simulink model "TEP_Final_NoScript"  (R2024a)
settings: Solver=FixedStepAuto  StartTime=0.0  StopTime=10  FixedStep=1/3600  RelTol=1e-3
model workspace (MAT data in the model file):
  AD : Simulink.Parameter (value not decoded)
  AG : Simulink.Parameter (value not decoded)
  AH : Simulink.Parameter (value not decoded)
  AV : Simulink.Parameter (value not decoded)
  AVP : Simulink.Parameter (value not decoded)
  BCHL : Simulink.Parameter (value not decoded)
  BCHV : Simulink.Parameter (value not decoded)
  BD : Simulink.Parameter (value not decoded)
  BG : Simulink.Parameter (value not decoded)
  BH : Simulink.Parameter (value not decoded)
  BVP : Simulink.Parameter (value not decoded)
  CD : Simulink.Parameter (value not decoded)
  CG : Simulink.Parameter (value not decoded)
  CH : Simulink.Parameter (value not decoded)
  CVP : Simulink.Parameter (value not decoded)
  XMW : Simulink.Parameter (value not decoded)
  XNS : Simulink.Parameter (value not decoded)
  XNSE : Simulink.Parameter (value not decoded)
symbols that are objects in the model workspace (value not decoded): AD, AG, AH, AV, AVP, BD, BG, BH, BVP, CD, CG, CH, CVP, XMW, XNS, XNSE
undefined symbols (not defined in the file or in its folder): magnitude, msgbox, SETPT, XMEAS, XMV
libraries: mylib x360, dspindex x28
(part 3 of 14)

== system TEP_Final_NoScript/Separator/Stream 10 ==
  XST(I,10) : Inport
  TST(10) : Inport  Port=2  PortDimensions=1
  VPOS(6) : Inport  Port=3  PortDimensions=1
  Bus Creator : BusCreator  Inputs=6
  FCM(I,10) Component molar flow of Stream 10 lb-mol/h : Product
  FTM(10) : Product  Inputs=*/
  HST(10) Molar Enthalpy of Stream 10 MBtu/lb-mol : Subsystem
  ITY : Constant
  Subsystem : Subsystem
  XMWS(10) Molecular weight of Stream 10 lb/lb-mol : Subsystem
  Properties of Stream 10 : Outport  VectorParamsAs1DForOutWhenUnconnected=off
  wires:
  XMWS(10) Molecular weight of Stream 10 lb/lb-mol/1(XMWS(10)) -> FTM(10)/2
  FTM(10)/1 -> Bus Creator/4, FCM(I,10) Component molar flow of Stream 10 lb-mol/h/2  "FTM(10)"
  ITY/1 -> Bus Creator/6, HST(10) Molar Enthalpy of Stream 10 MBtu/lb-mol/1(ITY)  "Phase"
  XST(I,10)/1 -> Bus Creator/1, FCM(I,10) Component molar flow of Stream 10 lb-mol/h/1, HST(10) Molar Enthalpy of Stream 10 MBtu/lb-mol/3(XST(I,I)), XMWS(10) Molecular weight of Stream 10 lb/lb-mol/1(XST(I,10))  "XST(I;10)"
  HST(10) Molar Enthalpy of Stream 10 MBtu/lb-mol/1("H ") -> Bus Creator/3  "HST(10)"
  TST(10)/1 -> Bus Creator/2, HST(10) Molar Enthalpy of Stream 10 MBtu/lb-mol/2(T)  "TST(10)"
  FCM(I,10) Component molar flow of Stream 10 lb-mol/h/1 -> Bus Creator/5  "FCM(I;10)"
  Bus Creator/1 -> Properties of Stream 10/1
  VPOS(6)/1 -> Subsystem/1(VPOS(6))
  Subsystem/1(Out1) -> FTM(10)/1

== system TEP_Final_NoScript/Separator/Stream 11 ==
  XST(I,11) : Inport  PortDimensions=8
  TST(11) : Inport  Port=2  PortDimensions=1
  VPOS(7) : Inport  Port=3
  "   " : Constant  Value=100
  Bus Creator : BusCreator  Inputs=7
  FCM(I,11) Component molar flow of Stream 11 lb-mol/h : Product
  FTM(11) : Product  Inputs=**/
  HST(10) Molar Enthalpy of Stream 10 MBtu/lb-mol : Subsystem
  ITY : Constant  Value=0
  PTSL Pressure of Liquid From Separator mmHg : Subsystem
  VRNG(7) : Constant  Value=1500
  Properties of Stream 11 : Outport  VectorParamsAs1DForOutWhenUnconnected=off
  wires:
  FTM(11)/1 -> Bus Creator/4, FCM(I,11) Component molar flow of Stream 11 lb-mol/h/2  "FTM(11)"
  ITY/1 -> Bus Creator/6, HST(10) Molar Enthalpy of Stream 10 MBtu/lb-mol/1(ITY)  "Phase"
  XST(I,11)/1 -> PTSL Pressure of Liquid From Separator mmHg/1(XLS), FCM(I,11) Component molar flow of Stream 11 lb-mol/h/1, Bus Creator/1, HST(10) Molar Enthalpy of Stream 10 MBtu/lb-mol/3(XST(I,I))  "XST(I;11)"
  HST(10) Molar Enthalpy of Stream 10 MBtu/lb-mol/1("H ") -> Bus Creator/3  "HST(11)"
  TST(11)/1 -> PTSL Pressure of Liquid From Separator mmHg/2(TCS), Bus Creator/2, HST(10) Molar Enthalpy of Stream 10 MBtu/lb-mol/2(T)  "TST(11)"
  VPOS(7)/1 -> FTM(11)/1
  FCM(I,11) Component molar flow of Stream 11 lb-mol/h/1 -> Bus Creator/5  "FCM(I;11)"
  VRNG(7)/1 -> FTM(11)/2
  "   "/1 -> FTM(11)/3
  Bus Creator/1 -> Properties of Stream 11/1
  PTSL Pressure of Liquid From Separator mmHg/1(PTSL) -> Bus Creator/7  "PTSL"

== system TEP_Final_NoScript/Separator/Stream 9 ==
  TST(9) : Inport
  XTS(I,9) : Inport  Port=2
  VPOS(5) : Inport  Port=3
  "  " : Product  Inputs=*/
  Bus Creator : BusCreator  Inputs=7
  FCM(I,9) Component molar flow of Stream 9 lb-mol/h : Product
  FTM(9) : Product  Inputs=*/
  HST(9) Molar Enthalpy of Stream 9 MBtu/lb-mol : Subsystem
  "HST(9) " : Sum
  ITY : Constant
  Subsystem : Subsystem
  XMWS(9) Molecular weight of Stream 9 lb/lb-mol : Subsystem
  Properties of Stream 9 : Outport  VectorParamsAs1DForOutWhenUnconnected=off
  wires:
  XTS(I,9)/1 -> XMWS(9) Molecular weight of Stream 9 lb/lb-mol/1(XST(I,9)), FCM(I,9) Component molar flow of Stream 9 lb-mol/h/2, Bus Creator/1, HST(9) Molar Enthalpy of Stream 9 MBtu/lb-mol/3(XST(I,I))  "XST(I;9)"
  TST(9)/1 -> Bus Creator/2, HST(9) Molar Enthalpy of Stream 9 MBtu/lb-mol/2(T)  "TST(9)"
  XMWS(9) Molecular weight of Stream 9 lb/lb-mol/1(XMWS(9)) -> Bus Creator/6, FTM(9)/2  "XMWS(9)"
  FTM(9)/1 -> Bus Creator/4, "  "/2, FCM(I,9) Component molar flow of Stream 9 lb-mol/h/1  "FTM(9)"
  [CPDH] -> "  "/1
  HST(9) Molar Enthalpy of Stream 9 MBtu/lb-mol/1("H ") -> "HST(9) "/1
  "  "/1 -> "HST(9) "/2
  "HST(9) "/1 -> Bus Creator/3  "HST(9)"
  FCM(I,9) Component molar flow of Stream 9 lb-mol/h/1 -> Bus Creator/5  "FCM(I;9)"
  Bus Creator/1 -> Properties of Stream 9/1
  VPOS(5)/1 -> Subsystem/1(VPOS(5))
  Subsystem/1("FLMS ") -> FTM(9)/1
  ITY/1 -> Bus Creator/7, HST(9) Molar Enthalpy of Stream 9 MBtu/lb-mol/1(ITY)  "Phase"

== system TEP_Final_NoScript/Separator/TCS Initial Temperature in Separator °C  ==
  UTLS : Inport
  ETS : Inport  Port=2  PortDimensions=1
  XLS : Inport  Port=3  PortDimensions=8
  "AG(I) Coefficient A to determine Enthalpy MBtu/lb·°F " : Constant  Value=AG
  "AH(I) Coefficient A to determine Enthalpy MBtu/lb·°F " : Constant  Value=AH
  AV(I) Coefficient AV to determine Enthalpy MBtu/lb : Constant  Value=AV
  BG(I) Coefficient B to determine Enthalpy MBtu/lb·°F² : Constant  Value=BG
  BH(I) Coefficient B to determine Enthalpy MBtu/lb·°F² : Constant  Value=BH
  CG(I) Coefficient C to determine Enthalpy MBtu/lb·°F³ : Constant  Value=CG
  CH(I) Coefficient C to determine Enthalpy MBtu/lb·°F³ : Constant  Value=CH
  Delay : Delay  DelayLength=1  InitialCondition=0
  Display1 : Display
  ITY : Constant  Value=0
  MATLAB Function : MATLAB Function  TreatAsAtomicUnit=on
  "XMW(I) Molecular weight of components lb/lb-mol " : Constant  Value=XMW
  TCS : Outport  PortDimensions=1  VectorParamsAs1DForOutWhenUnconnected=off
  wires:
  MATLAB Function/1(TCS) -> Delay/1, TCS/1
  Delay/1 -> MATLAB Function/13("TCS ")
  "AG(I) Coefficient A to determine Enthalpy MBtu/lb·°F "/1 -> MATLAB Function/4(AG)
  AV(I) Coefficient AV to determine Enthalpy MBtu/lb/1 -> MATLAB Function/7(AV)
  MATLAB Function/2(J) -> Display1/1
  ETS/1 -> MATLAB Function/10(ETS)
  CH(I) Coefficient C to determine Enthalpy MBtu/lb·°F³/1 -> MATLAB Function/3(CH)
  UTLS/1 -> MATLAB Function/11(UTLS)
  ITY/1 -> MATLAB Function/12(ITY)
  "XMW(I) Molecular weight of components lb/lb-mol "/1 -> MATLAB Function/8(XMW)
  XLS/1 -> MATLAB Function/9(XLS)
  "AH(I) Coefficient A to determine Enthalpy MBtu/lb·°F "/1 -> MATLAB Function/1(AH)
  CG(I) Coefficient C to determine Enthalpy MBtu/lb·°F³/1 -> MATLAB Function/6(CG)
  BH(I) Coefficient B to determine Enthalpy MBtu/lb·°F²/1 -> MATLAB Function/2(BH)
  BG(I) Coefficient B to determine Enthalpy MBtu/lb·°F²/1 -> MATLAB Function/5(BG)

== system TEP_Final_NoScript/Separator/Total Vapour Component Holdup in Separator ==
  XVS : Inport
  VVS : Inport  Port=2
  Display9 : Display
  RG Universal Gas Constant ft³·mmHg/K·lb-mol : Constant  Value=998.9
  TKS Temperature in Separator K : Sum
  To Convert °C to K : Constant  Value=273.15
  "UCVS(I) Vapour Component Holdup in Separator lb-mol  " : Product  Inputs=**
  UTVS Total Vapour Component Holdup in Reactor lb-mol : Product  Inputs=**//
  wires:
  UTVS Total Vapour Component Holdup in Reactor lb-mol/1 -> "UCVS(I) Vapour Component Holdup in Separator lb-mol  "/1
  VVS/1 -> UTVS Total Vapour Component Holdup in Reactor lb-mol/2
  [PTS] -> UTVS Total Vapour Component Holdup in Reactor lb-mol/1
  XVS/1 -> "UCVS(I) Vapour Component Holdup in Separator lb-mol  "/2
  "UCVS(I) Vapour Component Holdup in Separator lb-mol  "/1 -> Display9/1
  RG Universal Gas Constant ft³·mmHg/K·lb-mol/1 -> UTVS Total Vapour Component Holdup in Reactor lb-mol/3
  TKS Temperature in Separator K/1 -> UTVS Total Vapour Component Holdup in Reactor lb-mol/4
  [TCS] -> TKS Temperature in Separator K/1
  To Convert °C to K/1 -> TKS Temperature in Separator K/2

== system TEP_Final_NoScript/Separator/Vapour Component Fraction in Separator ==
  PPS : Inport
  Bus Creator2 : BusCreator  Inputs=8
  Bus Selector1 : BusSelector  OutputSignals=PPS(1),PPS(2),PPS(3),PPS(4),PPS(5),PPS(6),PPS(7),PPS(8)
  XVS(1) : Product  Inputs=*/
  XVS(2) : Product  Inputs=*/
  XVS(3) : Product  Inputs=*/
  XVS(4) : Product  Inputs=*/
  XVS(5) : Product  Inputs=*/
  XVS(6) : Product  Inputs=*/
  XVS(7) : Product  Inputs=*/
  XVS(8) : Product  Inputs=*/
  XVS : Outport  PortDimensions=8  VectorParamsAs1DForOutWhenUnconnected=off
  wires:
  XVS(1)/1 -> Bus Creator2/1  "XVS(1)"
  Bus Selector1/5 -> XVS(5)/1  "<PPS(5)>"
  Bus Selector1/7 -> XVS(7)/1  "<PPS(7)>"
  Bus Selector1/6 -> XVS(6)/1  "<PPS(6)>"
  XVS(8)/1 -> Bus Creator2/8  "XVS(8)"
  Bus Selector1/8 -> XVS(8)/1  "<PPS(8)>"
  XVS(2)/1 -> Bus Creator2/2  "XVS(2)"
  [PTS] -> XVS(8)/2, XVS(7)/2, XVS(6)/2, XVS(5)/2, XVS(4)/2, XVS(3)/2, XVS(2)/2, XVS(1)/2
  Bus Selector1/2 -> XVS(2)/1  "<PPS(2)>"
  XVS(7)/1 -> Bus Creator2/7  "XVS(7)"
  Bus Selector1/4 -> XVS(4)/1  "<PPS(4)>"
  Bus Creator2/1 -> XVS/1
  XVS(4)/1 -> Bus Creator2/4  "XVS(4)"
  XVS(6)/1 -> Bus Creator2/6  "XVS(6)"
  Bus Selector1/3 -> XVS(3)/1  "<PPS(3)>"
  XVS(5)/1 -> Bus Creator2/5  "XVS(5)"
  PPS/1 -> Bus Selector1/1
  Bus Selector1/1 -> XVS(1)/1  "<PPS(1)>"
  XVS(3)/1 -> Bus Creator2/3  "XVS(3)"

== system TEP_Final_NoScript/Separator/Volume of Separator ==
  UTLS : Inport  PortDimensions=1
  XLS : Inport  Port=2  PortDimensions=8
  "DLS Molar Density of Liquids in Reactor lb-mol/ft³    " : Subsystem
  "VLS Liquid Volume in Separator ft³ " : Product  Inputs=*/
  VTS Total Volume of Separator ft³ : Constant  Value=3500
  VVS Vapour Volume in Separator ft³ : Sum  Inputs=+-
  VVS : Outport  VectorParamsAs1DForOutWhenUnconnected=off
  VLS : Outport  Port=2  VectorParamsAs1DForOutWhenUnconnected=off
  tag scope: DLS=global
  wires:
  "VLS Liquid Volume in Separator ft³ "/1 -> VLS/1, VVS Vapour Volume in Separator ft³/2
  VVS Vapour Volume in Separator ft³/1 -> VVS/1
  UTLS/1 -> "VLS Liquid Volume in Separator ft³ "/1
  VTS Total Volume of Separator ft³/1 -> VVS Vapour Volume in Separator ft³/1
  "DLS Molar Density of Liquids in Reactor lb-mol/ft³    "/1("DLS ") -> [DLS], "VLS Liquid Volume in Separator ft³ "/2
  XLS/1 -> "DLS Molar Density of Liquids in Reactor lb-mol/ft³    "/1(XLS)
  [TCS] -> "DLS Molar Density of Liquids in Reactor lb-mol/ft³    "/2(TCS)

== system TEP_Final_NoScript/Shut Down Procedure/Reactor Level to High ==
  VLR : Inport
  Assertion : Assertion  AssertionFailFcn=disp(sprintf('\nSimulation stoped.')), msgbox({'Plant Shutdown';'Reactor Level to High'}, 'Shutdown','error')  StopWhenAssertionFail=off
  Assertion block : mylib/Assertion block  SystemSampleTime=-1  VariantActivationTime=update diagram  AllowFlexibleInterface=on  Latency=0  AutoFrameSizeCalculation=off
      settings: SourceProductName=TEP Library
  Constant : Constant  Value=24
  Constant1 : Constant  Value=35.145
  Divide : Product  Inputs=*/
  Relational Operator : RelationalOperator  Operator=>  OutDataTypeStr=boolean  RndMeth=Simplest  InputSameDT=off
  ISD : Outport  VectorParamsAs1DForOutWhenUnconnected=off
  wires:
  Relational Operator/1 -> ISD/1, Assertion block/1
  Constant/1 -> Relational Operator/2
  Divide/1 -> Relational Operator/1
  VLR/1 -> Divide/1
  Constant1/1 -> Divide/2
  Assertion block/1 -> Assertion/1

== system TEP_Final_NoScript/Shut Down Procedure/Reactor Level to Low ==
  VLR : Inport
  Assertion : Assertion  AssertionFailFcn=disp(sprintf('\nSimulation stoped.')), msgbox({'Plant Shutdown';'Reactor Level to Low'}, 'Shutdown','error')  StopWhenAssertionFail=off
  Assertion block : mylib/Assertion block  SystemSampleTime=-1  VariantActivationTime=update diagram  AllowFlexibleInterface=on  Latency=0  AutoFrameSizeCalculation=off
      settings: SourceProductName=TEP Library
  Constant : Constant  Value=2
  Constant1 : Constant  Value=35.145
  Divide : Product  Inputs=*/
  Relational Operator : RelationalOperator  Operator=<  OutDataTypeStr=boolean  RndMeth=Simplest  InputSameDT=off
  ISD : Outport  VectorParamsAs1DForOutWhenUnconnected=off
  wires:
  Relational Operator/1 -> ISD/1, Assertion block/1
  Constant/1 -> Relational Operator/2
  Divide/1 -> Relational Operator/1
  VLR/1 -> Divide/1
  Constant1/1 -> Divide/2
  Assertion block/1 -> Assertion/1

== system TEP_Final_NoScript/Shut Down Procedure/Reactor Presssure to High ==
  " " : Sum  Inputs=+-
  "    " : Constant  Value=760
  "       " : Constant  Value=101.325
  Assertion : Assertion  AssertionFailFcn=disp(sprintf('\nSimulation stoped.')), msgbox({'Plant Shutdown';'Reactor Pressure to High'}, 'Shutdown','error')  StopWhenAssertionFail=off
  Assertion block : mylib/Assertion block  SystemSampleTime=-1  VariantActivationTime=update diagram  AllowFlexibleInterface=on  Latency=0  AutoFrameSizeCalculation=off
      settings: SourceProductName=TEP Library
  Constant : Constant  Value=3000
  Relational Operator : RelationalOperator  Operator=>  RndMeth=Simplest  InputSameDT=off
  XMEAS(7) : Product  Inputs=*/*
  ISD : Outport  VectorParamsAs1DForOutWhenUnconnected=off
  wires:
  XMEAS(7)/1 -> Relational Operator/1
  Relational Operator/1 -> ISD/1, Assertion block/1
  Constant/1 -> Relational Operator/2
  "       "/1 -> XMEAS(7)/3
  " "/1 -> XMEAS(7)/1
  [PTR] -> " "/1
  "    "/1 -> XMEAS(7)/2, " "/2
  Assertion block/1 -> Assertion/1

== system TEP_Final_NoScript/Shut Down Procedure/Reactor Temperature to High ==
  Assertion : Assertion  AssertionFailFcn=disp(sprintf('\nSimulation stoped.')), msgbox({'Plant Shutdown';'Reactor Temperature to High'}, 'Shutdown','error')  StopWhenAssertionFail=off
  Assertion block : mylib/Assertion block  SystemSampleTime=-1  VariantActivationTime=update diagram  AllowFlexibleInterface=on  Latency=0  AutoFrameSizeCalculation=off
      settings: SourceProductName=TEP Library
  Constant : Constant  Value=175
  Relational Operator : RelationalOperator  Operator=>  OutDataTypeStr=boolean  RndMeth=Simplest  InputSameDT=off
  ISD : Outport  VectorParamsAs1DForOutWhenUnconnected=off
  wires:
  [TCR] -> Relational Operator/1
  Relational Operator/1 -> ISD/1, Assertion block/1
  Constant/1 -> Relational Operator/2
  Assertion block/1 -> Assertion/1

== system TEP_Final_NoScript/Shut Down Procedure/Separator Level to High ==
  VLS : Inport
  Assertion : Assertion  AssertionFailFcn=disp(sprintf('\nSimulation stoped.')), msgbox({'Plant Shutdown';'Separator Level to High'}, 'Shutdown','error')  StopWhenAssertionFail=off
  Assertion block : mylib/Assertion block  SystemSampleTime=-1  VariantActivationTime=update diagram  AllowFlexibleInterface=on  Latency=0  AutoFrameSizeCalculation=off
      settings: SourceProductName=TEP Library
  Constant : Constant  Value=12
  Constant1 : Constant  Value=35.145
  Divide : Product  Inputs=*/
  Relational Operator : RelationalOperator  Operator=>  OutDataTypeStr=boolean  RndMeth=Simplest  InputSameDT=off
  ISD : Outport  VectorParamsAs1DForOutWhenUnconnected=off
  wires:
  Relational Operator/1 -> ISD/1, Assertion block/1
  Constant/1 -> Relational Operator/2
  Divide/1 -> Relational Operator/1
  VLS/1 -> Divide/1
  Constant1/1 -> Divide/2
  Assertion block/1 -> Assertion/1

== system TEP_Final_NoScript/Shut Down Procedure/Separator Level to Low ==
  VLS : Inport
  Assertion : Assertion  AssertionFailFcn=disp(sprintf('\nSimulation stoped.')), msgbox({'Plant Shutdown';'Separator Level to Low'}, 'Shutdown','error')  StopWhenAssertionFail=off
  Assertion block : mylib/Assertion block  SystemSampleTime=-1  VariantActivationTime=update diagram  AllowFlexibleInterface=on  Latency=0  AutoFrameSizeCalculation=off
      settings: SourceProductName=TEP Library
  Constant : Constant
  Constant1 : Constant  Value=35.145
  Divide : Product  Inputs=*/
  Relational Operator : RelationalOperator  Operator=<  OutDataTypeStr=boolean  RndMeth=Simplest  InputSameDT=off
  ISD : Outport  VectorParamsAs1DForOutWhenUnconnected=off
  wires:
  Relational Operator/1 -> ISD/1, Assertion block/1
  Constant/1 -> Relational Operator/2
  Divide/1 -> Relational Operator/1
  VLS/1 -> Divide/1
  Constant1/1 -> Divide/2
  Assertion block/1 -> Assertion/1

== system TEP_Final_NoScript/Shut Down Procedure/Stripper Level to High ==
  VLC : Inport
  Assertion : Assertion  AssertionFailFcn=disp(sprintf('\nSimulation stoped.')), msgbox({'Plant Shutdown';'Stripper Level to High'}, 'Shutdown','error')  StopWhenAssertionFail=off
  Assertion block : mylib/Assertion block  SystemSampleTime=-1  VariantActivationTime=update diagram  AllowFlexibleInterface=on  Latency=0  AutoFrameSizeCalculation=off
      settings: SourceProductName=TEP Library
  Constant : Constant  Value=8
  Constant1 : Constant  Value=35.145
  Divide : Product  Inputs=*/
  Relational Operator : RelationalOperator  Operator=>  OutDataTypeStr=boolean  RndMeth=Simplest  InputSameDT=off
  ISD : Outport  VectorParamsAs1DForOutWhenUnconnected=off
  wires:
  Relational Operator/1 -> ISD/1, Assertion block/1
  Constant/1 -> Relational Operator/2
  VLC/1 -> Divide/1
  Constant1/1 -> Divide/2
  Divide/1 -> Relational Operator/1
  Assertion block/1 -> Assertion/1

== system TEP_Final_NoScript/Shut Down Procedure/Stripper Level to Low ==
  VLC : Inport
  Assertion : Assertion  AssertionFailFcn=disp(sprintf('\nSimulation stoped.')), msgbox({'Plant Shutdown';'Stripper Level to Low'}, 'Shutdown','error')  StopWhenAssertionFail=off
  Assertion block : mylib/Assertion block  SystemSampleTime=-1  VariantActivationTime=update diagram  AllowFlexibleInterface=on  Latency=0  AutoFrameSizeCalculation=off
      settings: SourceProductName=TEP Library
  Constant : Constant
  Constant1 : Constant  Value=35.145
  Divide : Product  Inputs=*/
  Relational Operator : RelationalOperator  Operator=<  OutDataTypeStr=boolean  RndMeth=Simplest  InputSameDT=off
  ISD : Outport  VectorParamsAs1DForOutWhenUnconnected=off
  wires:
  Relational Operator/1 -> ISD/1, Assertion block/1
  Constant/1 -> Relational Operator/2
  Divide/1 -> Relational Operator/1
  VLC/1 -> Divide/1
  Constant1/1 -> Divide/2
  Assertion block/1 -> Assertion/1

== system TEP_Final_NoScript/Stripper/Heat transfer of stripper ==
  VPOS(9) : Inport
  "  " : Constant  Value=0
  Add : Sum
  Bus Selector : BusSelector  OutputSignals=signal1.TESUB8(9)
  Constant : Constant
  Constant2 : Constant  Value=100
  If : If  IfExpression=u1 < 100
  If Action Subsystem : Subsystem  TreatAsAtomicUnit=on
  If Action Subsystem1 : Subsystem  TreatAsAtomicUnit=on
  Merge : Merge
  Product : Product
  Subtract : Sum  Inputs=+-
  UAC : Product  Inputs=***/
  VRNG(9) : Constant  Value=0.03
  tag scope: QUC=global
  wires:
  Constant/1 -> Add/1
  Bus Selector/1 -> Add/2  "<TESUB8(9)>"
  VPOS(9)/1 -> UAC/1
  VRNG(9)/1 -> UAC/2
  Add/1 -> UAC/3
  Constant2/1 -> Subtract/1, UAC/4
  If/1 -> If Action Subsystem/Action
  Product/1 -> If Action Subsystem/1(In1)
  [TCC] -> Subtract/2, If/1
  If/2 -> If Action Subsystem1/Action
  "  "/1 -> If Action Subsystem1/1(In1)
  Subtract/1 -> Product/2
  UAC/1 -> Product/1
  If Action Subsystem/1(Out1) -> Merge/1
  If Action Subsystem1/1(Out1) -> Merge/2
  Merge/1 -> [QUC]
  [TESUB8] -> Bus Selector/1

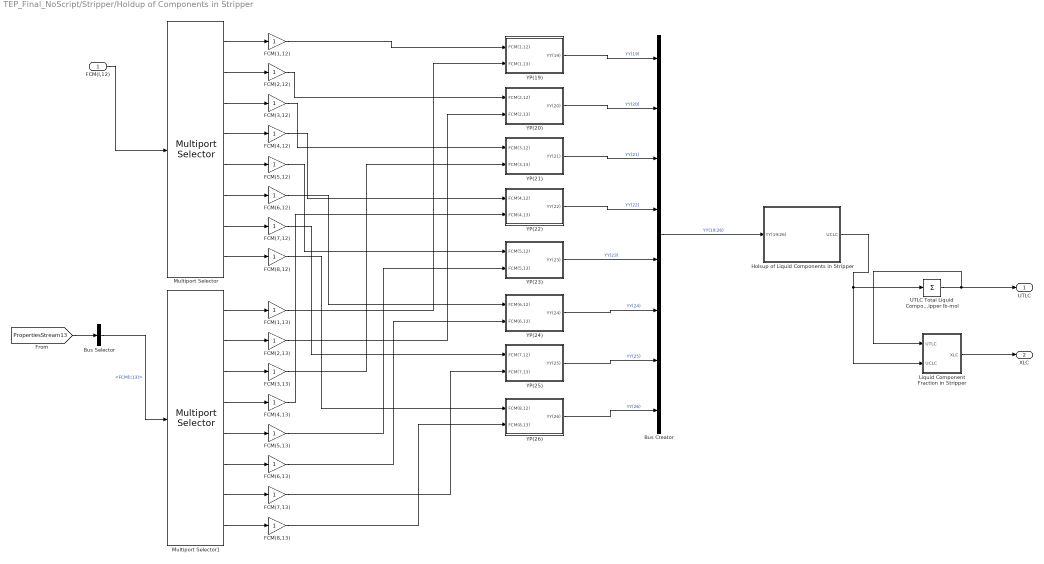
== system TEP_Final_NoScript/Stripper/Holdup of Components in Stripper ==
  "FCM(I,12) " : Inport
  Bus Creator : BusCreator  Inputs=8
  Bus Selector : BusSelector  OutputSignals=FCM(I;13)
  FCM(1,12) : Gain
  FCM(1,13) : Gain
  FCM(2,12) : Gain
  FCM(2,13) : Gain
  FCM(3,12) : Gain
  FCM(3,13) : Gain
  FCM(4,12) : Gain
  FCM(4,13) : Gain
  FCM(5,12) : Gain
  FCM(5,13) : Gain
  FCM(6,12) : Gain
  FCM(6,13) : Gain
  FCM(7,12) : Gain
  FCM(7,13) : Gain
  FCM(8,12) : Gain
  FCM(8,13) : Gain
  Holsup of Liquid Components in Stripper : Subsystem
  Liquid Component Fraction in Stripper : Subsystem
  Multiport Selector : dspindex/Multiport Selector  rowsOrCols=Rows  idxCellArray={ 1,2,3,4,5,6,7,8}  idxErrMode=Clip Index
  Multiport Selector1 : dspindex/Multiport Selector  rowsOrCols=Rows  idxCellArray={ 1,2,3,4,5,6,7,8}  idxErrMode=Clip Index
  UTLC Total Liquid Component holdup in Stripper lb-mol : Sum  Inputs=+
  YP(19) : Subsystem
  YP(20) : Subsystem
  YP(21) : Subsystem
  YP(22) : Subsystem
  YP(23) : Subsystem
  YP(24) : Subsystem
  YP(25) : Subsystem
  YP(26) : Subsystem
  UTLC : Outport  VectorParamsAs1DForOutWhenUnconnected=off
  XLC : Outport  Port=2  VectorParamsAs1DForOutWhenUnconnected=off
  wires:
  "FCM(I,12) "/1 -> Multiport Selector/1
  Multiport Selector/1 -> FCM(1,12)/1
  Multiport Selector/2 -> FCM(2,12)/1
  Multiport Selector/3 -> FCM(3,12)/1
  Multiport Selector/4 -> FCM(4,12)/1
  Multiport Selector/5 -> FCM(5,12)/1
  Multiport Selector/6 -> FCM(6,12)/1
  Multiport Selector/7 -> FCM(7,12)/1
  Multiport Selector/8 -> FCM(8,12)/1
  Multiport Selector1/1 -> FCM(1,13)/1
  Multiport Selector1/7 -> FCM(7,13)/1
  Multiport Selector1/2 -> FCM(2,13)/1
  Multiport Selector1/3 -> FCM(3,13)/1
  Multiport Selector1/5 -> FCM(5,13)/1
  Multiport Selector1/4 -> FCM(4,13)/1
  Multiport Selector1/8 -> FCM(8,13)/1
  Multiport Selector1/6 -> FCM(6,13)/1
  FCM(1,12)/1 -> YP(19)/1(FCM(1,12))
  YP(19)/1(YY(19)) -> Bus Creator/1  "YY(19)"
  YP(20)/1(YY(20)) -> Bus Creator/2  "YY(20)"
  YP(22)/1("YY(22)  ") -> Bus Creator/4  "YY(22)"
  YP(23)/1("YY(23)  ") -> Bus Creator/5  "YY(23)"
  YP(24)/1("YY(24)  ") -> Bus Creator/6  "YY(24)"
  YP(25)/1("YY(25)  ") -> Bus Creator/7  "YY(25)"
  YP(26)/1("YY(26)   ") -> Bus Creator/8  "YY(26)"
  FCM(1,13)/1 -> YP(19)/2(FCM(1,13))
  FCM(2,12)/1 -> YP(20)/1(FCM(2,12))
  FCM(3,12)/1 -> YP(21)/1(FCM(3,12))
  FCM(4,12)/1 -> YP(22)/1(FCM(4,12))
  FCM(5,12)/1 -> YP(23)/1(FCM(5,12))
  FCM(2,13)/1 -> YP(20)/2(FCM(2,13))
  FCM(3,13)/1 -> YP(21)/2(FCM(3,13))
  FCM(6,12)/1 -> YP(24)/1(FCM(6,12))
  FCM(7,12)/1 -> YP(25)/1(FCM(7,12))
  FCM(8,12)/1 -> YP(26)/1(FCM(8,12))
  FCM(4,13)/1 -> YP(22)/2(FCM(4,13))
  FCM(5,13)/1 -> YP(23)/2(FCM(5,13))
  FCM(6,13)/1 -> YP(24)/2(FCM(6,13))
  FCM(7,13)/1 -> YP(25)/2(FCM(7,13))
  FCM(8,13)/1 -> YP(26)/2(FCM(8,13))
  Bus Creator/1 -> Holsup of Liquid Components in Stripper/1(YY(19:26))  "YY(19:26)"
  Holsup of Liquid Components in Stripper/1(UCLC) -> Liquid Component Fraction in Stripper/2(UCLC), UTLC Total Liquid Component holdup in Stripper lb-mol/1
  YP(21)/1(YY(21)) -> Bus Creator/3  "YY(21)"
  UTLC Total Liquid Component holdup in Stripper lb-mol/1 -> Liquid Component Fraction in Stripper/1(UTLC), UTLC/1
  Liquid Component Fraction in Stripper/1(XLC) -> XLC/1
  [PropertiesStream13] -> Bus Selector/1
  Bus Selector/1 -> Multiport Selector1/1  "<FCM(I;13)>"

== system TEP_Final_NoScript/Stripper/Internal energy of stripper ==
  Properties of Stream 4 : Inport
  Properties of Stream 11 : Inport  Port=2
  Properties of Stream 5 : Inport  Port=3
  Add : Sum  Inputs=++--+
  Bus Selector : BusSelector  OutputSignals=HST(4),FTM(4)
  Bus Selector1 : BusSelector  OutputSignals=HST(11),FTM(11)
  Bus Selector2 : BusSelector  OutputSignals=HST(5),FTM(5)
  Bus Selector3 : BusSelector  OutputSignals=HST(13),FTM(13)
  Integration : mylib/Integration  SystemSampleTime=-1  VariantActivationTime=update diagram  AllowFlexibleInterface=on  Latency=0  AutoFrameSizeCalculation=off
      settings: SourceProductName=TEP Library
  Product{,1..3} (4 alike) : Product
  YY(27) : Constant  Value=0.3755297257
  "YY(27) " : Outport  VectorParamsAs1DForOutWhenUnconnected=off
  wires:
  Bus Selector/1 -> Product/1  "<HST(4)>"
  Bus Selector/2 -> Product/2  "<FTM(4)>"
  Bus Selector1/2 -> Product1/2  "<FTM(11)>"
  Bus Selector1/1 -> Product1/1  "<HST(11)>"
  Product/1 -> Add/1
  Product1/1 -> Add/2
  Integration/1 -> "YY(27) "/1
  YY(27)/1 -> Integration/2
  Add/1 -> Integration/1
  Bus Selector3/1 -> Product3/1  "<HST(13)>"
  Bus Selector2/2 -> Product2/2  "<FTM(5)>"
  Product2/1 -> Add/3
  Bus Selector3/2 -> Product3/2  "<FTM(13)>"
  Product3/1 -> Add/4
  Bus Selector2/1 -> Product2/1  "<HST(5)>"
  [QUC] -> Add/5
  Properties of Stream 4/1 -> Bus Selector/1
  Properties of Stream 11/1 -> Bus Selector1/1
  Properties of Stream 5/1 -> Bus Selector2/1
  [PropertiesStream13] -> Bus Selector3/1

== system TEP_Final_NoScript/Stripper/PTC Pressure of Liquid zone in stripper mmHg ==
  XLC : Inport
  TCC : Inport  Port=2
  Bus Creator1 : BusCreator  Inputs=8
  Demux : Demux  Outputs=8
  PPR(I) : Product
  PTR Total Pressure of Reactor mmHg : Sum  Inputs=+
  VPR Vapour Pressure mmHg : Subsystem
  PTC : Outport  PortDimensions=1  VectorParamsAs1DForOutWhenUnconnected=off
  wires:
  Demux/1 -> Bus Creator1/1  "PPR(1)"
  Demux/2 -> Bus Creator1/2  "PPR(2)"
  Demux/7 -> Bus Creator1/7  "PPR(7)"
  TCC/1 -> VPR Vapour Pressure mmHg/1(TCR)
  Demux/8 -> Bus Creator1/8  "PPR(8)"
  PPR(I)/1 -> Demux/1
  VPR Vapour Pressure mmHg/1(VPR) -> PPR(I)/2
  PTR Total Pressure of Reactor mmHg/1 -> PTC/1
  XLC/1 -> PPR(I)/1
  Bus Creator1/1 -> PTR Total Pressure of Reactor mmHg/1
  Demux/6 -> Bus Creator1/6  "PPR(6)"
  Demux/4 -> Bus Creator1/4  "PPR(4)"
  Demux/5 -> Bus Creator1/5  "PPR(5)"
  Demux/3 -> Bus Creator1/3  "PPR(3)"

== system TEP_Final_NoScript/Stripper/Position of Valve 8 % ==
  Bus Selector : BusSelector  OutputSignals=XMV(8)
  Bus Selector1 : BusSelector  OutputSignals=IDV(19)
  Control valve : mylib/Control valve  SystemSampleTime=-1  VariantActivationTime=update diagram  AllowFlexibleInterface=on  Latency=0  AutoFrameSizeCalculation=off
      settings: SourceProductName=TEP Library
  Divide : Product  Inputs=*/
  Integration : mylib/Integration  SystemSampleTime=-1  VariantActivationTime=update diagram  AllowFlexibleInterface=on  Latency=0  AutoFrameSizeCalculation=off
      settings: SourceProductName=TEP Library
  Subtract : Sum  Inputs=+-
  VTAU(8) : Constant  Value=5/3600
  YY(46) : Constant  Value=46.53415582
  "YY(46) " : Outport  PortDimensions=1  VectorParamsAs1DForOutWhenUnconnected=off
  wires:
  Integration/1 -> "YY(46) "/1, Subtract/2  "VPOS(8)"
  Subtract/1 -> Divide/1
  Control valve/1 -> Subtract/1
  VTAU(8)/1 -> Divide/2
  Divide/1 -> Integration/1
  YY(46)/1 -> Integration/2
  [XMV] -> Bus Selector/1
  Bus Selector/1 -> Control valve/1  "<XMV(8)>"
  [IDV] -> Bus Selector1/1
  Bus Selector1/1 -> Control valve/2  "<IDV(19)>"

== system TEP_Final_NoScript/Stripper/Position of Valve 9 % ==
  Bus Selector : BusSelector  OutputSignals=XMV(9)
  Bus Selector1 : BusSelector  OutputSignals=IDV(19)
  Control valve : mylib/Control valve  SystemSampleTime=-1  VariantActivationTime=update diagram  AllowFlexibleInterface=on  Latency=0  AutoFrameSizeCalculation=off
      settings: SourceProductName=TEP Library
  Divide : Product  Inputs=*/
  Integration : mylib/Integration  SystemSampleTime=-1  VariantActivationTime=update diagram  AllowFlexibleInterface=on  Latency=0  AutoFrameSizeCalculation=off
      settings: SourceProductName=TEP Library
  Subtract : Sum  Inputs=+-
  VTAU(9) : Constant  Value=120/3600
  YY(47) : Constant  Value=47.44573456
  "YY(47) " : Outport  PortDimensions=1  VectorParamsAs1DForOutWhenUnconnected=off
  wires:
  Integration/1 -> "YY(47) "/1, Subtract/2  "VPOS(9)"
  Subtract/1 -> Divide/1
  Control valve/1 -> Subtract/1
  VTAU(9)/1 -> Divide/2
  Divide/1 -> Integration/1
  YY(47)/1 -> Integration/2
  [XMV] -> Bus Selector/1
  Bus Selector/1 -> Control valve/1  "<XMV(9)>"
  Bus Selector1/1 -> Control valve/2  "<IDV(19)>"
  [IDV] -> Bus Selector1/1

== system TEP_Final_NoScript/Stripper/Split Fractions ==
  Bus Creator1 : BusCreator  Inputs=4
  SFR(1) : Constant  Value=0.99500
  SFR(2) : Constant  Value=0.99100
  SFR(3) : Constant  Value=0.99000
  Split fraction : Subsystem
  SFR : Outport  VectorParamsAs1DForOutWhenUnconnected=off
  wires:
  Bus Creator1/1 -> SFR/1
  SFR(2)/1 -> Bus Creator1/2
  Split fraction/1(SFR) -> Bus Creator1/4
  SFR(1)/1 -> Bus Creator1/1
  SFR(3)/1 -> Bus Creator1/3

== system TEP_Final_NoScript/Stripper/Stream 12 ==
  FCM(I,12) : Inport
  Bus Creator : BusCreator  Inputs=5
  Display : Display
  FTM(12) : Sum  Inputs=+
  Gain : Gain
  HST(12) Molar Enthalpy of Stream 12 MBtu/lb-mol : Subsystem
  ITY : Constant  Value=0
  XST(I,12) : Product  Inputs=*/
  wires:
  FTM(12)/1 -> XST(I,12)/2, Bus Creator/4  "FTM(12)"
  FCM(I,12)/1 -> XST(I,12)/1, Bus Creator/5, FTM(12)/1  "FCM(I;12)"
  XST(I,12)/1 -> Bus Creator/1, HST(12) Molar Enthalpy of Stream 12 MBtu/lb-mol/3(XST(I,I))  "XST(I;12)"
  [TCC] -> Gain/1
  Gain/1 -> Bus Creator/2, HST(12) Molar Enthalpy of Stream 12 MBtu/lb-mol/2(T)  "TST(12)"
  ITY/1 -> HST(12) Molar Enthalpy of Stream 12 MBtu/lb-mol/1(ITY)
  HST(12) Molar Enthalpy of Stream 12 MBtu/lb-mol/1("H ") -> Bus Creator/3  "HST(12)"
  Bus Creator/1 -> Display/1

== system TEP_Final_NoScript/Stripper/Stream 13 ==
  XST(I,13) : Inport  PortDimensions=8
  TST(13) : Inport  Port=2
  VPOS(8) : Inport  Port=3
  PTC : Inport  Port=4
  "   " : Constant  Value=100
  Bus Creator : BusCreator  Inputs=7
  FCM(I,13) Component molar flow of Stream 13 lb-mol/h : Product
  FTM(13) : Product  Inputs=**/
  HST(13) Molar Enthalpy of Stream 13 MBtu/lb-mol : Subsystem
  ITY : Constant  Value=0
  VRNG(8) : Constant  Value=1000
  Properties of Stream 13 : Outport  VectorParamsAs1DForOutWhenUnconnected=off
  wires:
  FTM(13)/1 -> Bus Creator/4, FCM(I,13) Component molar flow of Stream 13 lb-mol/h/2  "FTM(13)"
  ITY/1 -> Bus Creator/6, HST(13) Molar Enthalpy of Stream 13 MBtu/lb-mol/1(ITY)  "Phase"
  XST(I,13)/1 -> Bus Creator/1, FCM(I,13) Component molar flow of Stream 13 lb-mol/h/1, HST(13) Molar Enthalpy of Stream 13 MBtu/lb-mol/3(XST(I,I))  "XST(I;13)"
  HST(13) Molar Enthalpy of Stream 13 MBtu/lb-mol/1("H ") -> Bus Creator/3  "HST(13)"
  TST(13)/1 -> Bus Creator/2, HST(13) Molar Enthalpy of Stream 13 MBtu/lb-mol/2(T)  "TST(13)"
  VPOS(8)/1 -> FTM(13)/1
  FCM(I,13) Component molar flow of Stream 13 lb-mol/h/1 -> Bus Creator/5  "FCM(I;13)"
  VRNG(8)/1 -> FTM(13)/2
  "   "/1 -> FTM(13)/3
  Bus Creator/1 -> Properties of Stream 13/1
  PTC/1 -> Bus Creator/7  "PTC"

== system TEP_Final_NoScript/Stripper/Stream 5 ==
  FCM(I,5) : Inport
  Bus Creator : BusCreator  Inputs=7
  FTM(5) : Sum  Inputs=+
  HST(5) Molar Enthalpy of Stream 5 MBtu/lb-mol : Subsystem
  ITY : Constant
  XST(I,5) : Product  Inputs=*/
  Properties of Stream 5 : Outport  VectorParamsAs1DForOutWhenUnconnected=off
  tag scope: PropertiesStream5=global
  wires:
  FTM(5)/1 -> Bus Creator/4, XST(I,5)/2  "FTM(5)"
  FCM(I,5)/1 -> XST(I,5)/1, Bus Creator/5, FTM(5)/1  "FCM(I;5)"
  XST(I,5)/1 -> Bus Creator/1, HST(5) Molar Enthalpy of Stream 5 MBtu/lb-mol/3(XST(I,5))  "XST(I;5)"
  [TCC] -> Bus Creator/2, HST(5) Molar Enthalpy of Stream 5 MBtu/lb-mol/2(TST(5))  "TST(5)"
  ITY/1 -> Bus Creator/6, HST(5) Molar Enthalpy of Stream 5 MBtu/lb-mol/1(ITY)  "Phase"
  HST(5) Molar Enthalpy of Stream 5 MBtu/lb-mol/1("H ") -> Bus Creator/3  "HST(5)"
  Bus Creator/1 -> [PropertiesStream5], Properties of Stream 5/1
  [PTV] -> Bus Creator/7

== system TEP_Final_NoScript/Stripper/TCC Initial Temperature in Stripper °C  ==
  UTLC : Inport  PortDimensions=1
  ETC : Inport  Port=2  PortDimensions=1
  XLC : Inport  Port=3  PortDimensions=8
  "AG(I) Coefficient A to determine Enthalpy MBtu/lb·°F " : Constant  Value=[3.411e-6;0.3799e-6;0.2491e-6;0.3567e-6;0.3463e-6;0.393e-6;0.17e-6;0.15e-6]
  "AH(I) Coefficient A to determine Enthalpy MBtu/lb·°F " : Constant  Value=[1e-6;1e-6;1e-6;0.96e-6;0.573e-6;0.652e-6;0.515e-6;0.471e-6]
  AV(I) Coefficient AV to determine Enthalpy MBtu/lb : Constant  Value=[1e-6;1e-6;1e-6;86.7e-6;160e-6;160e-6;225e-6;209e-6]
  BG(I) Coefficient B to determine Enthalpy MBtu/lb·°F² : Constant  Value=[7.18e-10;1.08e-9;1.36e-11;8.51e-10;8.96e-10;1.02e-9;0;0]
  BH(I) Coefficient B to determine Enthalpy MBtu/lb·°F² : Constant  Value=[0;0;0;8.7e-9;2.41e-9;2.18e-9;5.65e-10;8.7e-10]
  CG(I) Coefficient C to determine Enthalpy MBtu/lb·°F³ : Constant  Value=[6e-13;-3.98e-13;-3.93e-14;-3.12e-13;-3.27e-13;-3.12e-13;0;0]
  CH(I) Coefficient C to determine Enthalpy MBtu/lb·°F³ : Constant  Value=[0;0;0;4.81e-11;1.82e-11;1.94e-11;3.82e-12;2.62e-12]
  Delay : Delay  DelayLength=1  InitialCondition=0
  Display1 : Display
  ITY : Constant  Value=0
  MATLAB Function : MATLAB Function  TreatAsAtomicUnit=on
  "XMW(I) Molecular weight of components lb/lb-mol " : Constant  Value=[2;25.4;28;32;46;48;62;76]
  TCC : Outport  PortDimensions=1  VectorParamsAs1DForOutWhenUnconnected=off
  wires:
  MATLAB Function/1(TCC) -> Delay/1, TCC/1
  Delay/1 -> MATLAB Function/13("TCC ")
  "AG(I) Coefficient A to determine Enthalpy MBtu/lb·°F "/1 -> MATLAB Function/4(AG)
  AV(I) Coefficient AV to determine Enthalpy MBtu/lb/1 -> MATLAB Function/7(AV)
  MATLAB Function/2(J) -> Display1/1
  ETC/1 -> MATLAB Function/10(ETC)
  CH(I) Coefficient C to determine Enthalpy MBtu/lb·°F³/1 -> MATLAB Function/3(CH)
  UTLC/1 -> MATLAB Function/11(UTLC)
  ITY/1 -> MATLAB Function/12(ITY)
  "XMW(I) Molecular weight of components lb/lb-mol "/1 -> MATLAB Function/8(XMW)
  XLC/1 -> MATLAB Function/9(XLC)
  "AH(I) Coefficient A to determine Enthalpy MBtu/lb·°F "/1 -> MATLAB Function/1(AH)
  CG(I) Coefficient C to determine Enthalpy MBtu/lb·°F³/1 -> MATLAB Function/6(CG)
  BH(I) Coefficient B to determine Enthalpy MBtu/lb·°F²/1 -> MATLAB Function/2(BH)
  BG(I) Coefficient B to determine Enthalpy MBtu/lb·°F²/1 -> MATLAB Function/5(BG)

== system TEP_Final_NoScript/Stripper/Volume of Stripper ==
  UTLC : Inport  PortDimensions=1
  XLC : Inport  Port=2  PortDimensions=8
  "DLC Molar Density of Liquids in Stripper lb-mol/ft³    " : Subsystem
  "VLC Liquid Volume in Stripper ft³ " : Product  Inputs=*/
  tag scope: DLC=global, VLC=global
  wires:
  "DLC Molar Density of Liquids in Stripper lb-mol/ft³    "/1("DLC ") -> [DLC], "VLC Liquid Volume in Stripper ft³ "/2
  XLC/1 -> "DLC Molar Density of Liquids in Stripper lb-mol/ft³    "/1(XLC)
  "VLC Liquid Volume in Stripper ft³ "/1 -> [VLC]
  [TCC] -> "DLC Molar Density of Liquids in Stripper lb-mol/ft³    "/2(TCC)
  UTLC/1 -> "VLC Liquid Volume in Stripper ft³ "/1

== system TEP_Final_NoScript/Subsystem/Braatz ==
  XMEAS : Inport
  " " : Subsystem  mask{Parameter1=XMV(1), Parameter2=XMEAS(2), SETPT1=3664.0, GAIN1=1.0, SI1=3, HIGH1=5811, Parameter1_copy=SETPT(1), Parameter2_copy=XMEAS(26), SETPT14=6.8820, GAIN14=8.3, TAUI14=3168.0/3600, SI14=360, HIGH14=100}
      mask prompts: Parameter1 "Manipulated Variable"; Parameter2 "Process Variable"; SETPT1 "Setpoint"; GAIN1 "Controller Gain"; SI1 "Sampling Interval"; HIGH1 "High Limit"; Parameter1_copy "Manipulated Variable"; Parameter2_copy "Process Variable"; SETPT14 "Setpoint"; GAIN14 "Controller Gain"; TAUI14 "Integral Time Constant"; SI14 "Sampling Interval"; HIGH14 "High Limit"
      mask DialogControl DescGroupVar Prompt: Control Variables
      mask DialogControl DescTextVar Prompt: Enter the control variables needed
      mask DialogControl ParameterGroupVar Prompt: Control 1
      mask DialogControl Container3 Prompt: Control 14
  " 1" : Subsystem  mask{Parameter1=XMV(2), Parameter2=XMEAS(3), SETPT2=4509.3, GAIN2=1.0, SI2=3, HIGH2=8354, Parameter1_copy=SETPT(2), Parameter2_copy=XMEAS(27), SETPT15=18.776, GAIN15=2.37, TAUI15=5069/3600, SI15=360, HIGH15=100}
      mask prompts: Parameter1 "Manipulated Variable"; Parameter2 "Process Variable"; SETPT2 "Setpoint"; GAIN2 "Controller Gain"; SI2 "Sampling Interval"; HIGH2 "High Limit"; Parameter1_copy "Manipulated Variable"; Parameter2_copy "Process Variable"; SETPT15 "Setpoint"; GAIN15 "Controller Gain"; TAUI15 "Integral Time Constant"; SI15 "Sampling Interval"; HIGH15 "High Limit"
      mask DialogControl DescGroupVar Prompt: Control Variables
      mask DialogControl DescTextVar Prompt: Enter the control variables needed
      mask DialogControl ParameterGroupVar Prompt: Control 2
      mask DialogControl Container3 Prompt: Control 15
  " 10" : Subsystem  mask{Parameter1=XMV(6), Parameter2=XMEAS(10), SETPT6=0.33712, GAIN6=1.22, SI6=3, HIGH6=1, Parameter1_copy=SETPT(6), Parameter2_copy=XMEAS(30), SETPT19=13.823, GAIN19=-83.2/5/3, TAUI19=6336/3600, SI19=360, HIGH19=26}
      mask prompts: Parameter1 "Manipulated Variable"; Parameter2 "Process Variable"; SETPT6 "Setpoint"; GAIN6 "Controller Gain"; SI6 "Sampling Interval"; HIGH6 "High Limit"; Parameter1_copy "Manipulated Variable"; Parameter2_copy "Process Variable"; SETPT19 "Setpoint"; GAIN19 "Controller Gain"; TAUI19 "Integral Time Constant"; SI19 "Sampling Interval"; HIGH19 "High Limit"
      mask DialogControl DescGroupVar Prompt: Control Variables
      mask DialogControl DescTextVar Prompt: Enter the control variables needed
      mask DialogControl ParameterGroupVar Prompt: Control 6
      mask DialogControl Container3 Prompt: Control 19
  " 2" : Subsystem  mask{Parameter1=XMV(3), Parameter2=XMEAS(1), SETPT3=0.25052, GAIN3=1.0, SI3=3, HIGH3=1.017, Parameter1_copy=SETPT(3), Parameter2_copy=XMEAS(23), SETPT13=32.188, GAIN13=18, TAUI13=3168.0/3600, SI13=360, HIGH13=100}
      mask prompts: Parameter1 "Manipulated Variable"; Parameter2 "Process Variable"; SETPT3 "Setpoint"; GAIN3 "Controller Gain"; SI3 "Sampling Interval"; HIGH3 "High Limit"; Parameter1_copy "Manipulated Variable"; Parameter2_copy "Process Variable"; SETPT13 "Setpoint"; GAIN13 "Controller Gain"; TAUI13 "Integral Time Constant"; SI13 "Sampling Interval"; HIGH13 "High Limit"
      mask DialogControl DescGroupVar Prompt: Control Variables
      mask DialogControl DescTextVar Prompt: Enter the control variables needed
      mask DialogControl ParameterGroupVar Prompt: Control 3
      mask DialogControl Container3 Prompt: Control 13
  " 3" : Subsystem  mask{Parameter1=XMV(4), Parameter2=XMEAS(4), SETPT4=9.3477, GAIN4=1.0, SI4=3, HIGH4=15.25, Parameter1_copy=SETPT(4), Parameter2_copy=XMEAS(8), SETPT17=75, GAIN17=11.1/10, TAUI17=3168.0/3600, SI17=3, HIGH17=50}
      mask prompts: Parameter1 "Manipulated Variable"; Parameter2 "Process Variable"; SETPT4 "Setpoint"; GAIN4 "Controller Gain"; SI4 "Sampling Interval"; HIGH4 "High Limit"; Parameter1_copy "Manipulated Variable"; Parameter2_copy "Process Variable"; SETPT17 "Setpoint"; GAIN17 "Controller Gain"; TAUI17 "Integral Time Constant"; SI17 "Sampling Interval"; HIGH17 "High Limit"
      mask DialogControl DescGroupVar Prompt: Control Variables
      mask DialogControl DescTextVar Prompt: Enter the control variables needed
      mask DialogControl ParameterGroupVar Prompt: Control 4
      mask DialogControl Container3 Prompt: Control 17
  " 4" : Subsystem  mask{Parameter1_copy=XMV(5), Parameter2_copy=XMEAS(5), SETPT5=26.902, GAIN5=-0.083, TAUI5=1/3600, SI5=3, HIGH5=53}
      mask prompts: Parameter1_copy "Manipulated Variable"; Parameter2_copy "Process Variable"; SETPT5 "Setpoint"; GAIN5 "Controller Gain"; TAUI5 "Integral Time Constant"; SI5 "Sampling Interval"; HIGH5 "High Limit"
      mask DialogControl DescGroupVar Prompt: Control Variables
      mask DialogControl DescTextVar Prompt: Enter the control variables needed
      mask DialogControl Container3 Prompt: Control 5
  " 5" : Subsystem  mask{Parameter1_copy=XMV(7), Parameter2_copy=XMEAS(12), SETPT7=50, GAIN7=-2.06, SI7=3, HIGH7=70}
      mask prompts: Parameter1_copy "Manipulated Variable"; Parameter2_copy "Process Variable"; SETPT7 "Setpoint"; GAIN7 "Controller Gain"; SI7 "Sampling Interval"; HIGH7 "High Limit"
      mask DialogControl DescGroupVar Prompt: Control Variables
      mask DialogControl DescTextVar Prompt: Enter the control variables needed
      mask DialogControl Container3 Prompt: Control 7
  " 6" : Subsystem  mask{Parameter1_copy=XMV(8), Parameter2_copy=XMEAS(15), SETPT8=50, GAIN8=-1.62, SI8=3, HIGH8=70}
      mask prompts: Parameter1_copy "Manipulated Variable"; Parameter2_copy "Process Variable"; SETPT8 "Setpoint"; GAIN8 "Controller Gain"; SI8 "Sampling Interval"; HIGH8 "High Limit"
      mask DialogControl DescGroupVar Prompt: Control Variables
      mask DialogControl DescTextVar Prompt: Enter the control variables needed
      mask DialogControl Container3 Prompt: Control 8
  " 7" : Subsystem  mask{Parameter1_copy=XMV(11), Parameter2_copy=XMEAS(17), SETPT11=22.949, GAIN11=1.09, TAUI11=2600/3600, SI11=3, HIGH11=46}
      mask prompts: Parameter1_copy "Manipulated Variable"; Parameter2_copy "Process Variable"; SETPT11 "Setpoint"; GAIN11 "Controller Gain"; TAUI11 "Integral Time Constant"; SI11 "Sampling Interval"; HIGH11 "High Limit"
      mask DialogControl DescGroupVar Prompt: Control Variables
      mask DialogControl DescTextVar Prompt: Enter the control variables needed
      mask DialogControl Container3 Prompt: Control 11
  " 8" : Subsystem  mask{Parameter1=XMV(10), Parameter2=XMEAS(21), SETPT10=94.599, GAIN10=-0.156*10, TAUI10=1452/3600, SI10=3, HIGH10=150, Parameter1_copy=SETPT(10), Parameter2_copy=XMEAS(9), SETPT18=120.4, GAIN18=2.83*10, TAUI18=982/3600, SI18=3, HIGH18=150}
      mask prompts: Parameter1 "Manipulated Variable"; Parameter2 "Process Variable"; SETPT10 "Setpoint"; GAIN10 "Controller Gain"; TAUI10 "Integral Time Constant"; SI10 "Sampling Interval"; HIGH10 "High Limit"; Parameter1_copy "Manipulated Variable"; Parameter2_copy "Process Variable"; SETPT18 "Setpoint"; GAIN18 "Controller Gain"; TAUI18 "Integral Time Constant"; SI18 "Sampling Interval"; HIGH18 "High Limit"
      mask DialogControl DescGroupVar Prompt: Control Variables
      mask DialogControl DescTextVar Prompt: Enter the control variables needed
      mask DialogControl ParameterGroupVar Prompt: Control 10
      mask DialogControl Container3 Prompt: Control 18
  " 9" : Subsystem  mask{Parameter1=XMV(9), Parameter2=XMEAS(19), SETPT9=230.31, GAIN9=0.41, SI9=3, HIGH9=460, Parameter1_copy=SETPT(9), Parameter2_copy=XMEAS(18), SETPT16=65.731, GAIN16=1.69/10, TAUI16=236/3600, SI16=3, HIGH16=130, Parameter1_copy_copy=SETPT(16), Parameter2_copy_copy=XMEAS(38), SETPT20=0.83570, GAIN20=-16.3/5, TAUI20=12408/3600, SI20=900, HIGH20=1.6}
      mask prompts: Parameter1 "Manipulated Variable"; Parameter2 "Process Variable"; SETPT9 "Setpoint"; GAIN9 "Controller Gain"; SI9 "Sampling Interval"; HIGH9 "High Limit"; Parameter1_copy "Manipulated Variable"; Parameter2_copy "Process Variable"; SETPT16 "Setpoint"; GAIN16 "Controller Gain"; TAUI16 "Integral Time Constant"; SI16 "Sampling Interval"; HIGH16 "High Limit"; Parameter1_copy_copy "Manipulated Variable"; Parameter2_copy_copy "Process Variable"; SETPT20 "Setpoint"; GAIN20 "Controller Gain"; TAUI20 "Integral Time Constant"; SI20 "Sampling Interval"; HIGH20 "High Limit"
      mask DialogControl DescGroupVar Prompt: Control Variables
      mask DialogControl DescTextVar Prompt: Enter the control variables needed
      mask DialogControl ParameterGroupVar Prompt: Control 9
      mask DialogControl Container3 Prompt: Control 16
      mask DialogControl Container3_copy Prompt: Control 20
  Bus Creator : BusCreator  Inputs=12
  Constant11 : Constant  Value=XMV12_0
  XMV : Outport  VectorParamsAs1DForOutWhenUnconnected=off
  wires:
  " "/1(XMV(1)) -> Bus Creator/1  "XMV(1)"
  " 1"/1(XMV(2)) -> Bus Creator/2  "XMV(2)"
  " 2"/1(XMV(3)) -> Bus Creator/3  "XMV(3)"
  " 3"/1(XMV(4)) -> Bus Creator/4  "XMV(4)"
  " 4"/1(XMV(5)) -> Bus Creator/5  "XMV(5)"
  " 10"/1(XMV(6)) -> Bus Creator/6  "XMV(6)"
  " 5"/1(XMV(7)) -> Bus Creator/7  "XMV(7)"
  " 6"/1(XMV(8)) -> Bus Creator/8  "XMV(8)"
  " 9"/1(XMV(9)) -> Bus Creator/9  "XMV(9)"
  " 8"/1(XMV(10)) -> Bus Creator/10  "XMV(10)"
  " 7"/1(XMV(11)) -> Bus Creator/11  "XMV(11)"
  Constant11/1 -> Bus Creator/12  "XMV(12)"
  Bus Creator/1 -> XMV/1
  XMEAS/1 -> " 5"/1(XMEAS), " 9"/1(XMEAS), " 8"/1(XMEAS), " 7"/1(XMEAS), " 6"/1(XMEAS), " 10"/1(XMEAS), " 4"/1(XMEAS), " 3"/1(XMEAS), " 2"/1(XMEAS), " 1"/1(XMEAS), " "/1(XMEAS)

== system TEP_Final_NoScript/Subsystem/If Action Subsystem ==
  In1 : Inport
  Action Port : ActionPort  ActionPortLabel=if(u1 == 1)
  Out1 : Outport  VectorParamsAs1DForOutWhenUnconnected=off
  wires:
  In1/1 -> Out1/1

== system TEP_Final_NoScript/Subsystem/If Action Subsystem1 ==
  In1 : Inport
  Action Port : ActionPort  ActionPortLabel=elseif(u2 == 1)
  Out1 : Outport  VectorParamsAs1DForOutWhenUnconnected=off
  wires:
  In1/1 -> Out1/1

== system TEP_Final_NoScript/Subsystem/If Action Subsystem2 ==
  In1 : Inport
  Action Port : ActionPort  ActionPortLabel=elseif( u3 == 1)
  Out1 : Outport  VectorParamsAs1DForOutWhenUnconnected=off
  wires:
  In1/1 -> Out1/1

== system TEP_Final_NoScript/Subsystem/Open loop ==
  Bus Creator : BusCreator  Inputs=12
  Constant : Constant  Value=XMV1_0
  Constant1 : Constant  Value=XMV2_0
  Constant10 : Constant  Value=XMV11_0
  Constant11 : Constant  Value=XMV12_0
  Constant2 : Constant  Value=XMV3_0
  Constant3 : Constant  Value=XMV4_0
  Constant4 : Constant  Value=XMV5_0
  Constant5 : Constant  Value=XMV6_0
  Constant6 : Constant  Value=XMV7_0
  Constant7 : Constant  Value=XMV8_0
  Constant8 : Constant  Value=XMV9_0
  Constant9 : Constant  Value=XMV10_0
  XMV : Outport  VectorParamsAs1DForOutWhenUnconnected=off
  wires:
  Constant5/1 -> Bus Creator/6  "XMV(6)"
  Constant1/1 -> Bus Creator/2  "XMV(2)"
  Constant4/1 -> Bus Creator/5  "XMV(5)"
  Constant3/1 -> Bus Creator/4  "XMV(4)"
  Constant2/1 -> Bus Creator/3  "XMV(3)"
  Constant11/1 -> Bus Creator/12  "XMV(12)"
  Constant10/1 -> Bus Creator/11  "XMV(11)"
  Constant/1 -> Bus Creator/1  "XMV(1)"
  Constant9/1 -> Bus Creator/10  "XMV(10)"
  Constant8/1 -> Bus Creator/9  "XMV(9)"
  Constant6/1 -> Bus Creator/7  "XMV(7)"
  Bus Creator/1 -> XMV/1
  Constant7/1 -> Bus Creator/8  "XMV(8)"

== system TEP_Final_NoScript/Subsystem/Ricker ==
  Bus Creator : BusCreator  Inputs=12
  Constant : Constant  Value=XMV1_0
  Constant1 : Constant  Value=XMV2_0
  Constant10 : Constant  Value=XMV11_0
  Constant11 : Constant  Value=XMV12_0
  Constant2 : Constant  Value=XMV3_0
  Constant3 : Constant  Value=XMV4_0
  Constant4 : Constant  Value=XMV5_0
  Constant5 : Constant  Value=XMV6_0
  Constant6 : Constant  Value=XMV7_0
  Constant7 : Constant  Value=XMV8_0
  Constant8 : Constant  Value=XMV9_0
  Constant9 : Constant  Value=XMV10_0
  XMV : Outport  VectorParamsAs1DForOutWhenUnconnected=off
  wires:
  Constant5/1 -> Bus Creator/6  "XMV(6)"
  Constant1/1 -> Bus Creator/2  "XMV(2)"
  Constant4/1 -> Bus Creator/5  "XMV(5)"
  Constant3/1 -> Bus Creator/4  "XMV(4)"
  Constant2/1 -> Bus Creator/3  "XMV(3)"
  Constant11/1 -> Bus Creator/12  "XMV(12)"
  Constant10/1 -> Bus Creator/11  "XMV(11)"
  Constant/1 -> Bus Creator/1  "XMV(1)"
  Constant9/1 -> Bus Creator/10  "XMV(10)"
  Constant8/1 -> Bus Creator/9  "XMV(9)"
  Constant6/1 -> Bus Creator/7  "XMV(7)"
  Bus Creator/1 -> XMV/1
  Constant7/1 -> Bus Creator/8  "XMV(8)"

== system TEP_Final_NoScript/Subsystem/Subsystem ==
  OPL : Inport
  B : Inport  Port=2
  R : Inport  Port=3
  Assertion : Assertion  AssertionFailFcn=|  StopWhenAssertionFail=off
      | set_param(bdroot,'SimulationCommand','stop'),
      | disp(sprintf('\nSimulation stoped.')), msgbox({'Simulation will not run';'More than one loop selected'}, 'Shutdown','error')
  Constant3 : Constant  Value=2
  Relational Operator : RelationalOperator  Operator=<  OutDataTypeStr=boolean  RndMeth=Simplest  InputSameDT=off
  Sum of Elements : Sum  Inputs=+++
  wires:
  Sum of Elements/1 -> Relational Operator/1
  R/1 -> Sum of Elements/3
  OPL/1 -> Sum of Elements/1
  Relational Operator/1 -> Assertion/1
  Constant3/1 -> Relational Operator/2
  B/1 -> Sum of Elements/2

== system TEP_Final_NoScript/Subsystem1/A and C feed stream ==
  Stream 4 : Inport
  Bus Creator : BusCreator  Inputs=4
  Bus Selector : BusSelector  OutputSignals=XMNSE(7),XMNSE(8)
  Bus Selector1 : BusSelector  OutputSignals=TST(4),XST(I;4)
  Bus Selector2 : BusSelector  OutputSignals=Stream 4
  Bus Selector3 : BusSelector  OutputSignals=signal1.XMEAS(4)
  Composition measurement mol% : Subsystem
  Constant : Constant  Value=1000
  Flow measurement in kg/h : Subsystem
  Pressure measurement in kPa : Subsystem
  Temperature measurement in C : Subsystem
  SMEAS 4 : Outport
  tag scope: SM4=global
  wires:
  Bus Selector1/1 -> Temperature measurement in C/1(T in celsius)  "<TST(4)>"
  Temperature measurement in C/1(SMEAST) -> Bus Creator/1
  [XMNSE] -> Bus Selector/1
  Bus Selector/1 -> Temperature measurement in C/2(XMNSE)  "<XMNSE(7)>"
  Bus Selector/2 -> Pressure measurement in kPa/2(XMNSE)  "<XMNSE(8)>"
  Stream 4/1 -> Bus Selector1/1
  Bus Selector1/2 -> Flow measurement in kg/h/2(XST), Composition measurement mol%/1(XST)  "<XST(I;4)>"
  Constant/1 -> Pressure measurement in kPa/1("P in mm Hg ")
  Pressure measurement in kPa/1(SMEASP) -> Bus Creator/2
  Flow measurement in kg/h/1("SMEASF ") -> Bus Creator/3  "SMEASF"
  Composition measurement mol%/1(SMEASX) -> Bus Creator/4
  Bus Creator/1 -> [SM4], SMEAS 4/1
  [XMNSE2] -> Bus Selector2/1
  Bus Selector2/1 -> Composition measurement mol%/2(XMNSE)  "<Stream 4>"
  [XMEAS] -> Bus Selector3/1
  Bus Selector3/1 -> Flow measurement in kg/h/1(XMEAS in kscmh)  "<XMEAS(4)>"
